simulink model "OrientationAnimationModel"  (R2021b)
settings: Solver=FixedStepAuto  StartTime=0.0  StopTime=1000  FixedStep=.01  RelTol=1e-3
model workspace (MAT data in the model file):
  orbit_altitude = 450000
  r_earth = 6378100
  vel_init = 7640
libraries: matrix_library x5, vrlib x4, aerolibutil x1
settings Model: Creator=Ian Lee  LastModifiedBy=Ian Lee

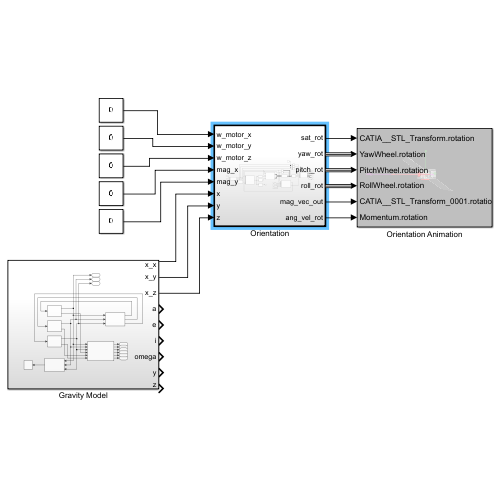
[thumbnail: Simulink's stored preview of the top-level diagram]
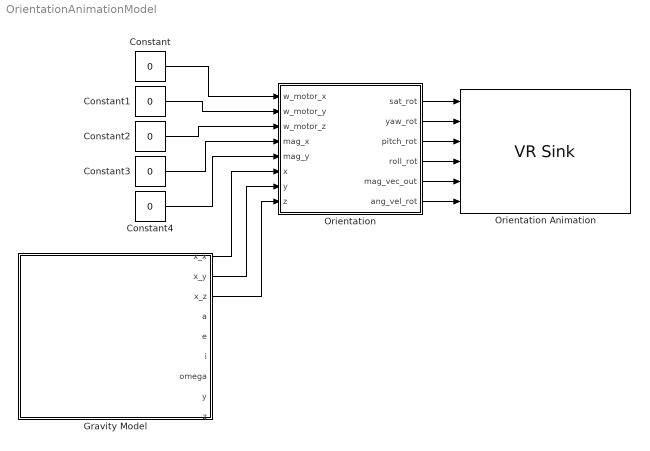
== system OrientationAnimationModel ==
  Constant{,1..4} (5 alike) : Constant  Value=0
  Gravity Model : Subsystem
  Orientation : Subsystem  TreatAsAtomicUnit=on
  Orientation Animation : vrlib/VR Sink  InstantiateOnLoad=on  SampleTime=.02  ViewEnable=on  RemoteChange=off  RemoteView=off  FieldsWritten=CATIA__STL_Transform.rotation.4.1.1.double#YawWheel.rotation.4.1.1.double#PitchWheel.rotation.4.1.1.double#RollWheel.rotation.4.1.1.double#CATIA__STL_Transform_0001.rotation.4.1.1.double#Momentum.rotation.4.1.1.double  WorldFileName=SatVR.x3d  AutoView=off  VideoDimensions=[]  AllowVariableSize=off  FigureProperties="{'Position', 'Name', 'Viewpoint', 'CameraBound', 'CameraDirection', 'CameraPosition', 'CameraUpVector', 'ZoomFactor', 'Antialiasing', 'Headlight', 'Lighting', 'NavPanel', 'Sound', 'StatusBar', 'Stereo3D', 'Stereo3DCameraOffset', 'Stereo3DHIT', 'ToolBar', 'Textures', 'Transparency', 'Triad', 'Wireframe', 'NavZones', 'NavMode', 'NavSpeed', 'CaptureFileFormat', 'CaptureFileName', 'Record2DCompressMethod', 'Record2DCompressQuality', 'Record2D', 'Record2DFileName', 'Record2DFPS'; [1.9340000000000000e+03  -2.3500000000000000e+02   1.0450000000000000e+03   5.1800000000000000e+02], '', '', 'on', [9.3422561981923258e-01  -2.9372272322992476e-01   2.0235971222811577e-01], [-9.5587776533600538e+02   2.6133093944556913e+02  -2.2202783758914998e+02], [2.5834757823765275e-01   9.4839129528426602e-01   1.8387626232948465e-01], [1.0000000000000000e+00], 'on', 'on', 'on', 'halfbar', 'on', 'on', 'off', [1.0000000149011612e-01], [0.0000000000000000e+00], 'on', 'on', 'on', 'none', 'off', 'on', 'examine', 'normal', 'tif', '%f_anim_%n.tif', 'auto', [7.5000000000000000e+01], 'off', '%f_anim_%n.avi', 'auto'}"
  wires:
  Orientation/1(sat_rot) -> Orientation Animation/1
  Orientation/2(yaw_rot) -> Orientation Animation/2
  Orientation/3(pitch_rot) -> Orientation Animation/3
  Orientation/4(roll_rot) -> Orientation Animation/4
  Orientation/5(mag_vec_out) -> Orientation Animation/5
  Orientation/6(ang_vel_rot) -> Orientation Animation/6
  Constant4/1 -> Orientation/5(mag_y)
  Constant3/1 -> Orientation/4(mag_x)
  Constant2/1 -> Orientation/3(w_motor_z)
  Constant1/1 -> Orientation/2(w_motor_y)
  Constant/1 -> Orientation/1(w_motor_x)
  Gravity Model/1(x_x) -> Orientation/6(x)
  Gravity Model/2(x_y) -> Orientation/7(y)
  Gravity Model/3(x_z) -> Orientation/8(z)

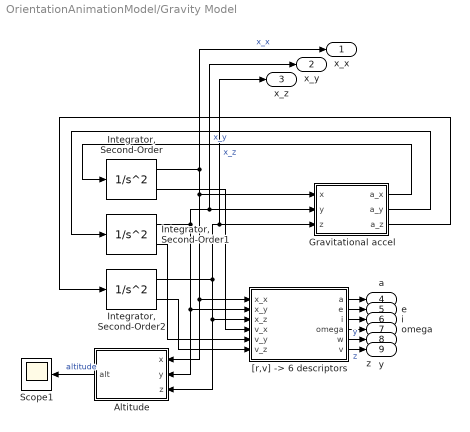
== system OrientationAnimationModel/Gravity Model ==
  Altitude : MATLAB Function  TreatAsAtomicUnit=on
  Gravitational accel : MATLAB Function  TreatAsAtomicUnit=on
  "Integrator, Second-Order" : SecondOrderIntegrator  ICX=0  ICDXDT=5500
  "Integrator, Second-Order1" : SecondOrderIntegrator  ICX=r_earth + orbit_altitude  ICDXDT=0
  "Integrator, Second-Order2" : SecondOrderIntegrator  ICDXDT=5300
  Scope1 : Scope
  "[r,v] -> 6 descriptors" : MATLAB Function  TreatAsAtomicUnit=on
  x_x : Outport
  x_y : Outport  Port=2
  x_z : Outport  Port=3
  a : Outport  Port=4
  e : Outport  Port=5
  i : Outport  Port=6
  omega : Outport  Port=7
  y : Outport  Port=8
  z : Outport  Port=9
  wires:
  Altitude/1(alt) -> Scope1/1  "altitude"
  "Integrator, Second-Order"/1 -> x_x/1, "[r,v] -> 6 descriptors"/1(x_x), Altitude/1(x), Gravitational accel/1(x)  "x_x"
  Gravitational accel/3(a_z) -> "Integrator, Second-Order2"/1
  Gravitational accel/1(a_x) -> "Integrator, Second-Order"/1
  "Integrator, Second-Order1"/1 -> "[r,v] -> 6 descriptors"/2(x_y), Altitude/2(y), x_y/1, Gravitational accel/2(y)  "x_y"
  "Integrator, Second-Order"/2 -> "[r,v] -> 6 descriptors"/4(v_x)
  Gravitational accel/2(a_y) -> "Integrator, Second-Order1"/1
  "Integrator, Second-Order2"/1 -> "[r,v] -> 6 descriptors"/3(x_z), Altitude/3(z), x_z/1, Gravitational accel/3(z)  "x_z"
  "Integrator, Second-Order2"/2 -> "[r,v] -> 6 descriptors"/6(v_z)
  "[r,v] -> 6 descriptors"/4(omega) -> omega/1
  "Integrator, Second-Order1"/2 -> "[r,v] -> 6 descriptors"/5(v_y)
  "[r,v] -> 6 descriptors"/1(a) -> a/1
  "[r,v] -> 6 descriptors"/2(e) -> e/1
  "[r,v] -> 6 descriptors"/5(w) -> y/1  "y"
  "[r,v] -> 6 descriptors"/6(v) -> z/1  "z"
  "[r,v] -> 6 descriptors"/3(i) -> i/1

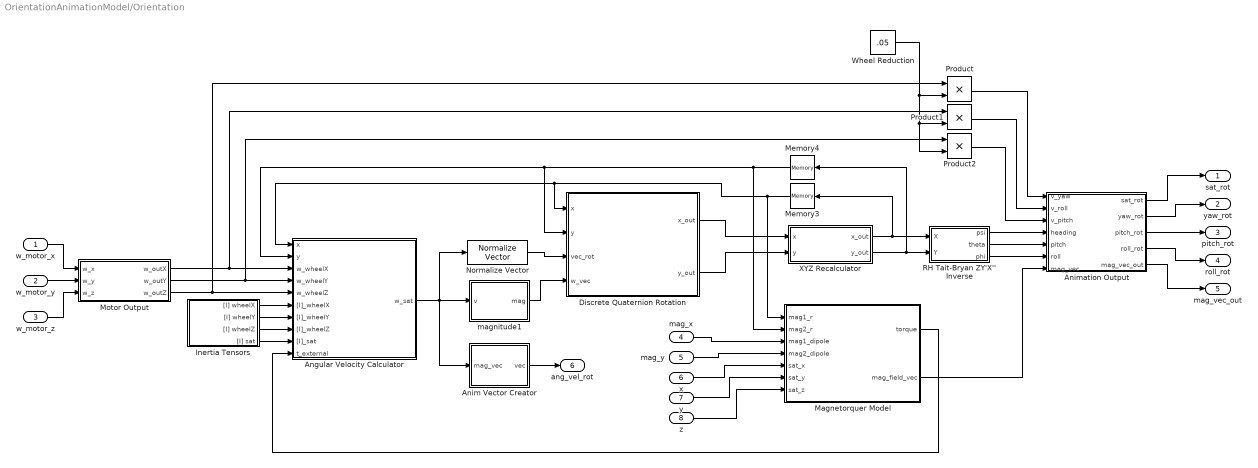
== system OrientationAnimationModel/Orientation ==
  w_motor_x : Inport
  w_motor_y : Inport  Port=2
  w_motor_z : Inport  Port=3
  mag_x : Inport  Port=4
  mag_y : Inport  Port=5
  x : Inport  Port=6
  y : Inport  Port=7
  z : Inport  Port=8
  Angular Velocity Calculator : Subsystem  TreatAsAtomicUnit=on
  Anim Vector Creator : MATLAB Function  TreatAsAtomicUnit=on
  Animation Output : Subsystem  TreatAsAtomicUnit=on
  Discrete Quaternion Rotation : Subsystem  TreatAsAtomicUnit=on
      mask Display: image('C:\Users\benml\Downloads\imageMas.png'); % Use "Edit Image" on toolstrip to change.
  Inertia Tensors : Subsystem  TreatAsAtomicUnit=on
  Magnetorquer Model : Subsystem  TreatAsAtomicUnit=on
  Memory3 : Memory  InitialCondition=[1,0,0]
  Memory4 : Memory  InitialCondition=[0,1,0]
  Motor Output : Subsystem  TreatAsAtomicUnit=on
  Normalize Vector : vrlib/Utilities/Normalize Vector  maxzero=0
  Product : Product
  Product1 : Product
  Product2 : Product
  RH Tait-Bryan ZY'X'' Inverse : MATLAB Function  TreatAsAtomicUnit=on
  Wheel Reduction : Constant  Value=.05
  XYZ Recalculator : Subsystem  TreatAsAtomicUnit=on
  magnitude1 : MATLAB Function  TreatAsAtomicUnit=on
  sat_rot : Outport
  yaw_rot : Outport  Port=2
  pitch_rot : Outport  Port=3
  roll_rot : Outport  Port=4
  mag_vec_out : Outport  Port=5
  ang_vel_rot : Outport  Port=6
  wires:
  Magnetorquer Model/1(torque) -> Angular Velocity Calculator/10(t_external)
  XYZ Recalculator/1(x_out) -> Memory3/1, RH Tait-Bryan ZY'X'' Inverse/1(X)
  RH Tait-Bryan ZY'X'' Inverse/2(theta) -> Animation Output/5(pitch)
  RH Tait-Bryan ZY'X'' Inverse/1(psi) -> Animation Output/4(heading)
  Discrete Quaternion Rotation/1(x_out) -> XYZ Recalculator/1(x)
  Product2/1 -> Animation Output/3(v_pitch)
  Discrete Quaternion Rotation/2(y_out) -> XYZ Recalculator/2(y)
  Product1/1 -> Animation Output/2(v_roll)
  Animation Output/2(yaw_rot) -> yaw_rot/1
  Animation Output/3(pitch_rot) -> pitch_rot/1
  Motor Output/1(w_outX) -> Angular Velocity Calculator/3(w_wheelX), Product1/1
  XYZ Recalculator/2(y_out) -> RH Tait-Bryan ZY'X'' Inverse/2(Y), Memory4/1
  RH Tait-Bryan ZY'X'' Inverse/3(phi) -> Animation Output/6(roll)
  Motor Output/3(w_outZ) -> Angular Velocity Calculator/5(w_wheelZ), Product/1
  Motor Output/2(w_outY) -> Product2/1, Angular Velocity Calculator/4(w_wheelY)
  Animation Output/1(sat_rot) -> sat_rot/1
  Product/1 -> Animation Output/1(v_yaw)
  Memory3/1 -> Magnetorquer Model/1(mag1_r), Discrete Quaternion Rotation/1(x), Angular Velocity Calculator/1(x)
  Animation Output/5(mag_vec_out) -> mag_vec_out/1
  Memory4/1 -> Magnetorquer Model/2(mag2_r), Discrete Quaternion Rotation/2(y), Angular Velocity Calculator/2(y)
  Animation Output/4(roll_rot) -> roll_rot/1
  z/1 -> Magnetorquer Model/7(sat_z)
  y/1 -> Magnetorquer Model/6(sat_y)
  x/1 -> Magnetorquer Model/5(sat_x)
  w_motor_y/1 -> Motor Output/2(w_y)
  w_motor_x/1 -> Motor Output/1(w_x)
  w_motor_z/1 -> Motor Output/3(w_z)
  mag_x/1 -> Magnetorquer Model/3(mag1_dipole)
  mag_y/1 -> Magnetorquer Model/4(mag2_dipole)
  Inertia Tensors/1("[I] wheelX") -> Angular Velocity Calculator/6("[I]_wheelX")
  Inertia Tensors/2("[I] wheelY") -> Angular Velocity Calculator/7("[I]_wheelY")
  Inertia Tensors/3("[I] wheelZ") -> Angular Velocity Calculator/8("[I]_wheelZ")
  Inertia Tensors/4("[I] sat") -> Angular Velocity Calculator/9("[I]_sat")
  Angular Velocity Calculator/1(w_sat) -> Normalize Vector/1, Anim Vector Creator/1(mag_vec), magnitude1/1(v)
  Normalize Vector/1 -> Discrete Quaternion Rotation/3(vec_rot)
  magnitude1/1(mag) -> Discrete Quaternion Rotation/4(w_vec)
  Anim Vector Creator/1(vec) -> ang_vel_rot/1
  Magnetorquer Model/2(mag_field_vec) -> Animation Output/7(mag_vec)
  Wheel Reduction/1 -> Product2/2, Product1/2, Product/2

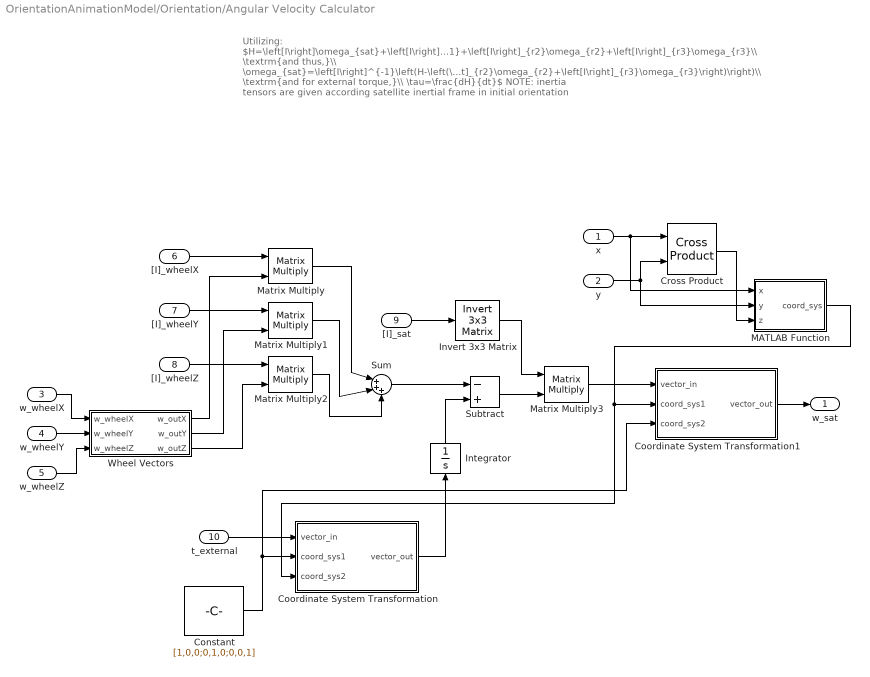
== system OrientationAnimationModel/Orientation/Angular Velocity Calculator ==
  note: Utilizing:
      | $H=\left[I\right]\omega_{sat}+\left[I\right]_{r1}\omega_{r1}+\left[I\right]_{r2}\omega_{r2}+\left[I\right]_{r3}\omega_{r3}\\ \textrm{and thus,}\\ \omega_{sat}=\left[I\right]^{-1}\left(H-\left(\left[I\right]_{r1}\omega_{r1}+\left[I\right]_{r2}\omega_{r2}+\left[I\right]_{r3}\omega_{r3}\right)\right)\\ \textrm{and for external torque,}\\ \tau=\frac{dH}{dt}$
      |
      | NOTE: inertia tensors are given according satellite inertial frame in initial orientation
  x : Inport
  y : Inport  Port=2
  w_wheelX : Inport  Port=3
  w_wheelY : Inport  Port=4
  w_wheelZ : Inport  Port=5
  "[I]_wheelX" : Inport  Port=6
  "[I]_wheelY" : Inport  Port=7
  "[I]_wheelZ" : Inport  Port=8
  "[I]_sat" : Inport  Port=9
  t_external : Inport  Port=10
  Constant : Constant  Value=[1,0,0;0,1,0;0,0,1]
  Coordinate System Transformation : MATLAB Function  TreatAsAtomicUnit=on
  Coordinate System Transformation1 : MATLAB Function  TreatAsAtomicUnit=on
  Cross Product : matrix_library/Cross Product
      settings: SourceProductBaseCode=SL
  Integrator : Integrator
  Invert 3x3 Matrix : aerolibutil/Invert  3x3 Matrix
  MATLAB Function : MATLAB Function  TreatAsAtomicUnit=on
  Matrix Multiply{,1..3} (4 alike) : Product  Multiplication=Matrix(*)
  Subtract : Sum  Inputs=-+
  Sum : Sum  Inputs=|+++
  Wheel Vectors : Subsystem  TreatAsAtomicUnit=on
  w_sat : Outport
  wires:
  "[I]_sat"/1 -> Invert 3x3 Matrix/1
  w_wheelX/1 -> Wheel Vectors/1(w_wheelX)
  w_wheelY/1 -> Wheel Vectors/2(w_wheelY)
  w_wheelZ/1 -> Wheel Vectors/3(w_wheelZ)
  "[I]_wheelX"/1 -> Matrix Multiply/1
  "[I]_wheelY"/1 -> Matrix Multiply1/1
  "[I]_wheelZ"/1 -> Matrix Multiply2/1
  Wheel Vectors/1(w_outX) -> Matrix Multiply/2
  Wheel Vectors/2(w_outY) -> Matrix Multiply1/2
  Wheel Vectors/3(w_outZ) -> Matrix Multiply2/2
  Matrix Multiply1/1 -> Sum/2
  Matrix Multiply2/1 -> Sum/3
  Matrix Multiply/1 -> Sum/1
  Invert 3x3 Matrix/1 -> Matrix Multiply3/1
  x/1 -> MATLAB Function/1(x), Cross Product/1
  y/1 -> MATLAB Function/2(y), Cross Product/2
  Cross Product/1 -> MATLAB Function/3(z)
  MATLAB Function/1(coord_sys) -> Coordinate System Transformation/3(coord_sys2), Coordinate System Transformation1/2(coord_sys1)
  Subtract/1 -> Matrix Multiply3/2
  t_external/1 -> Coordinate System Transformation/1(vector_in)
  Sum/1 -> Subtract/1
  Constant/1 -> Coordinate System Transformation/2(coord_sys1), Coordinate System Transformation1/3(coord_sys2)
  Matrix Multiply3/1 -> Coordinate System Transformation1/1(vector_in)
  Coordinate System Transformation1/1(vector_out) -> w_sat/1
  Coordinate System Transformation/1(vector_out) -> Integrator/1
  Integrator/1 -> Subtract/2

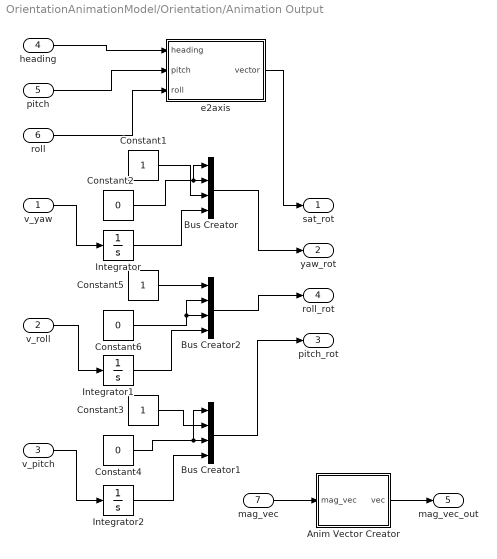
== system OrientationAnimationModel/Orientation/Animation Output ==
  v_yaw : Inport
  v_roll : Inport  Port=2
  v_pitch : Inport  Port=3
  heading : Inport  Port=4
  pitch : Inport  Port=5
  roll : Inport  Port=6
  mag_vec : Inport  Port=7
  Anim Vector Creator : MATLAB Function  TreatAsAtomicUnit=on
  Bus Creator : BusCreator  Inputs=4
  Bus Creator1 : BusCreator  Inputs=4
  Bus Creator2 : BusCreator  Inputs=4
  Constant1 : Constant
  Constant2 : Constant  Value=0
  Constant3 : Constant
  Constant4 : Constant  Value=0
  Constant5 : Constant
  Constant6 : Constant  Value=0
  Integrator : Integrator
  Integrator1 : Integrator
  Integrator2 : Integrator
  e2axis : MATLAB Function  TreatAsAtomicUnit=on
  sat_rot : Outport
  yaw_rot : Outport  Port=2
  pitch_rot : Outport  Port=3
  roll_rot : Outport  Port=4
  mag_vec_out : Outport  Port=5
  wires:
  Constant6/1 -> Bus Creator2/2, Bus Creator2/3
  Constant5/1 -> Bus Creator2/1
  Constant1/1 -> Bus Creator/3
  Constant3/1 -> Bus Creator1/2
  Constant2/1 -> Bus Creator/1, Bus Creator/2
  Constant4/1 -> Bus Creator1/1, Bus Creator1/3
  heading/1 -> e2axis/1(heading)
  pitch/1 -> e2axis/2(pitch)
  roll/1 -> e2axis/3(roll)
  e2axis/1(vector) -> sat_rot/1
  v_yaw/1 -> Integrator/1
  v_roll/1 -> Integrator1/1
  v_pitch/1 -> Integrator2/1
  Bus Creator/1 -> yaw_rot/1
  Bus Creator2/1 -> roll_rot/1
  Bus Creator1/1 -> pitch_rot/1
  Integrator/1 -> Bus Creator/4
  Integrator1/1 -> Bus Creator2/4
  Integrator2/1 -> Bus Creator1/4
  mag_vec/1 -> Anim Vector Creator/1(mag_vec)
  Anim Vector Creator/1(vec) -> mag_vec_out/1

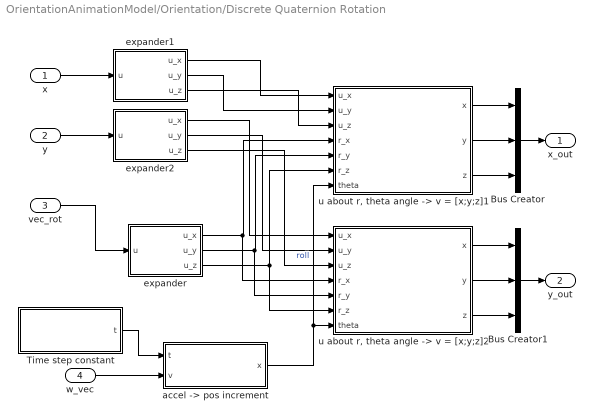
== system OrientationAnimationModel/Orientation/Discrete Quaternion Rotation ==
  x : Inport
  y : Inport  Port=2
  vec_rot : Inport  Port=3
  w_vec : Inport  Port=4
  Bus Creator : BusCreator  Inputs=3
  Bus Creator1 : BusCreator  Inputs=3
  Time step constant : Subsystem  TreatAsAtomicUnit=on
  "accel -> pos increment" : Subsystem  TreatAsAtomicUnit=on
  expander : MATLAB Function  TreatAsAtomicUnit=on
  expander1 : MATLAB Function  TreatAsAtomicUnit=on
  expander2 : MATLAB Function  TreatAsAtomicUnit=on
  "u about r, theta angle -> v = [x;y;z]1" : Subsystem  TreatAsAtomicUnit=on
  "u about r, theta angle -> v = [x;y;z]2" : Subsystem  TreatAsAtomicUnit=on
  x_out : Outport
  y_out : Outport  Port=2
  wires:
  x/1 -> expander1/1(u)
  vec_rot/1 -> expander/1(u)
  expander1/1(u_x) -> "u about r, theta angle -> v = [x;y;z]1"/1(u_x)
  expander1/2(u_y) -> "u about r, theta angle -> v = [x;y;z]1"/2(u_y)
  expander1/3(u_z) -> "u about r, theta angle -> v = [x;y;z]1"/3(u_z)
  expander/1(u_x) -> "u about r, theta angle -> v = [x;y;z]2"/4(r_x), "u about r, theta angle -> v = [x;y;z]1"/4(r_x)
  expander/2(u_y) -> "u about r, theta angle -> v = [x;y;z]2"/5(r_y), "u about r, theta angle -> v = [x;y;z]1"/5(r_y)
  expander/3(u_z) -> "u about r, theta angle -> v = [x;y;z]1"/6(r_z), "u about r, theta angle -> v = [x;y;z]2"/6(r_z)
  expander2/1(u_x) -> "u about r, theta angle -> v = [x;y;z]2"/1(u_x)
  expander2/2(u_y) -> "u about r, theta angle -> v = [x;y;z]2"/2(u_y)
  expander2/3(u_z) -> "u about r, theta angle -> v = [x;y;z]2"/3(u_z)
  y/1 -> expander2/1(u)
  Time step constant/1(t) -> "accel -> pos increment"/1(t)
  "accel -> pos increment"/1(x) -> "u about r, theta angle -> v = [x;y;z]1"/7(theta), "u about r, theta angle -> v = [x;y;z]2"/7(theta)  "roll"
  w_vec/1 -> "accel -> pos increment"/2("v ")
  "u about r, theta angle -> v = [x;y;z]1"/1(x) -> Bus Creator/1
  "u about r, theta angle -> v = [x;y;z]1"/2(y) -> Bus Creator/2
  "u about r, theta angle -> v = [x;y;z]1"/3(z) -> Bus Creator/3
  Bus Creator/1 -> x_out/1
  Bus Creator1/1 -> y_out/1
  "u about r, theta angle -> v = [x;y;z]2"/2(y) -> Bus Creator1/2
  "u about r, theta angle -> v = [x;y;z]2"/1(x) -> Bus Creator1/1
  "u about r, theta angle -> v = [x;y;z]2"/3(z) -> Bus Creator1/3

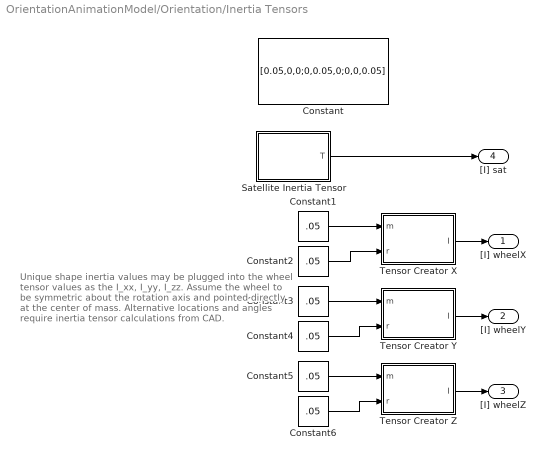
== system OrientationAnimationModel/Orientation/Inertia Tensors ==
  note: Unique shape inertia values may be plugged into
      | the wheel tensor values as the I_xx, I_yy, I_zz. Assume
      | the wheel to be symmetric about the rotation axis
      | and pointed directly at the center of mass.
      | Alternative locations and angles require inertia
      | tensor calculations from CAD.
  Constant : Constant  Value=[0.05,0,0;0,0.05,0;0,0,0.05]
  Constant{1..6} (6 alike) : Constant  Value=.05
  Satellite Inertia Tensor : MATLAB Function  TreatAsAtomicUnit=on
  Tensor Creator X : MATLAB Function  TreatAsAtomicUnit=on
  Tensor Creator Y : MATLAB Function  TreatAsAtomicUnit=on
  Tensor Creator Z : MATLAB Function  TreatAsAtomicUnit=on
  "[I] wheelX" : Outport
  "[I] wheelY" : Outport  Port=2
  "[I] wheelZ" : Outport  Port=3
  "[I] sat" : Outport  Port=4
  wires:
  Constant2/1 -> Tensor Creator X/2(r)
  Constant1/1 -> Tensor Creator X/1(m)
  Constant4/1 -> Tensor Creator Y/2(r)
  Constant3/1 -> Tensor Creator Y/1(m)
  Constant6/1 -> Tensor Creator Z/2(r)
  Constant5/1 -> Tensor Creator Z/1(m)
  Tensor Creator Y/1(I) -> "[I] wheelY"/1
  Tensor Creator X/1(I) -> "[I] wheelX"/1
  Tensor Creator Z/1(I) -> "[I] wheelZ"/1
  Satellite Inertia Tensor/1(T) -> "[I] sat"/1

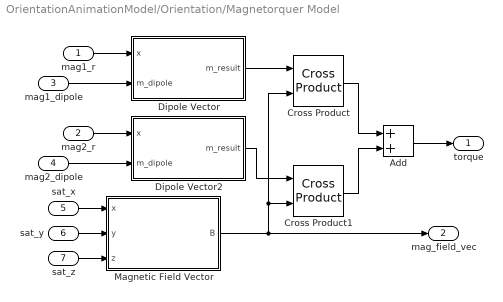
== system OrientationAnimationModel/Orientation/Magnetorquer Model ==
  mag1_r : Inport
  mag2_r : Inport  Port=2
  mag1_dipole : Inport  Port=3
  mag2_dipole : Inport  Port=4
  sat_x : Inport  Port=5
  sat_y : Inport  Port=6
  sat_z : Inport  Port=7
  Add : Sum
  Cross Product : matrix_library/Cross Product
      settings: SourceProductBaseCode=SL
  Cross Product1 : matrix_library/Cross Product
      settings: SourceProductBaseCode=SL
  Dipole Vector : MATLAB Function  TreatAsAtomicUnit=on
  Dipole Vector2 : MATLAB Function  TreatAsAtomicUnit=on
  Magnetic Field Vector : MATLAB Function  TreatAsAtomicUnit=on
  torque : Outport
  mag_field_vec : Outport  Port=2
  wires:
  Cross Product1/1 -> Add/2
  mag1_dipole/1 -> Dipole Vector/2(m_dipole)
  Cross Product/1 -> Add/1
  Dipole Vector2/1(m_result) -> Cross Product1/1
  sat_x/1 -> Magnetic Field Vector/1(x)
  sat_z/1 -> Magnetic Field Vector/3(z)
  sat_y/1 -> Magnetic Field Vector/2(y)
  Magnetic Field Vector/1(B) -> mag_field_vec/1, Cross Product/2, Cross Product1/2
  mag2_dipole/1 -> Dipole Vector2/2(m_dipole)
  Dipole Vector/1(m_result) -> Cross Product/1
  Add/1 -> torque/1
  mag2_r/1 -> Dipole Vector2/1(x)
  mag1_r/1 -> Dipole Vector/1(x)

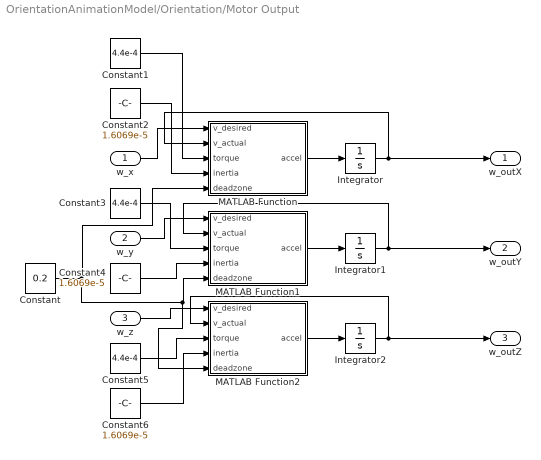
== system OrientationAnimationModel/Orientation/Motor Output ==
  w_x : Inport
  w_y : Inport  Port=2
  w_z : Inport  Port=3
  Constant : Constant  Value=0.2
  Constant1 : Constant  Value=4.4e-4
  Constant2 : Constant  Value=1.6069e-5
  Constant3 : Constant  Value=4.4e-4
  Constant4 : Constant  Value=1.6069e-5
  Constant5 : Constant  Value=4.4e-4
  Constant6 : Constant  Value=1.6069e-5
  Integrator : Integrator
  Integrator1 : Integrator
  Integrator2 : Integrator
  MATLAB Function : MATLAB Function  TreatAsAtomicUnit=on
  MATLAB Function1 : MATLAB Function  TreatAsAtomicUnit=on
  MATLAB Function2 : MATLAB Function  TreatAsAtomicUnit=on
  w_outX : Outport
  w_outY : Outport  Port=2
  w_outZ : Outport  Port=3
  wires:
  Constant1/1 -> MATLAB Function/3(torque)
  Constant2/1 -> MATLAB Function/4(inertia)
  MATLAB Function/1(accel) -> Integrator/1
  Integrator/1 -> MATLAB Function/2(v_actual), w_outX/1
  w_x/1 -> MATLAB Function/1(v_desired)
  Constant3/1 -> MATLAB Function1/3(torque)
  Constant4/1 -> MATLAB Function1/4(inertia)
  MATLAB Function1/1(accel) -> Integrator1/1
  Integrator1/1 -> w_outY/1, MATLAB Function1/2(v_actual)
  w_y/1 -> MATLAB Function1/1(v_desired)
  Constant5/1 -> MATLAB Function2/3(torque)
  Constant6/1 -> MATLAB Function2/4(inertia)
  MATLAB Function2/1(accel) -> Integrator2/1
  Integrator2/1 -> MATLAB Function2/2(v_actual), w_outZ/1
  w_z/1 -> MATLAB Function2/1(v_desired)
  Constant/1 -> MATLAB Function2/5(deadzone), MATLAB Function1/5(deadzone), MATLAB Function/5(deadzone)

== system OrientationAnimationModel/Orientation/XYZ Recalculator ==
  x : Inport
  y : Inport  Port=2
  Cross Product : matrix_library/Cross Product
      settings: SourceProductBaseCode=SL
  Cross Product1 : matrix_library/Cross Product
      settings: SourceProductBaseCode=SL
  Normalize Vector : vrlib/Utilities/Normalize Vector  maxzero=0
  Normalize Vector1 : vrlib/Utilities/Normalize Vector  maxzero=0
  x_out : Outport
  y_out : Outport  Port=2
  wires:
  x/1 -> Normalize Vector1/1
  y/1 -> y_out/1, Cross Product1/1, Normalize Vector/1
  Normalize Vector1/1 -> Cross Product/1
  Normalize Vector/1 -> Cross Product/2
  Cross Product/1 -> Cross Product1/2
  Cross Product1/1 -> x_out/1

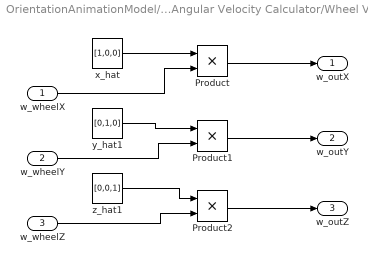
== system OrientationAnimationModel/Orientation/Angular Velocity Calculator/Wheel Vectors ==
  w_wheelX : Inport
  w_wheelY : Inport  Port=2
  w_wheelZ : Inport  Port=3
  Product : Product
  Product1 : Product
  Product2 : Product
  x_hat : Constant  Value=[1,0,0]
  y_hat1 : Constant  Value=[0,1,0]
  z_hat1 : Constant  Value=[0,0,1]
  w_outX : Outport
  w_outY : Outport  Port=2
  w_outZ : Outport  Port=3
  wires:
  x_hat/1 -> Product/1
  w_wheelX/1 -> Product/2
  y_hat1/1 -> Product1/1
  z_hat1/1 -> Product2/1
  w_wheelY/1 -> Product1/2
  w_wheelZ/1 -> Product2/2
  Product/1 -> w_outX/1
  Product1/1 -> w_outY/1
  Product2/1 -> w_outZ/1

== system OrientationAnimationModel/Orientation/Discrete Quaternion Rotation/Time step constant ==
  Clock : Clock
  Memory : Memory  InitialCondition=0.1
  Subtract : Sum  Inputs=+-
  t : Outport
  wires:
  Clock/1 -> Memory/1, Subtract/1
  Memory/1 -> Subtract/2
  Subtract/1 -> t/1

== system OrientationAnimationModel/Orientation/Discrete Quaternion Rotation/accel -> pos increment ==
  t : Inport
  "v " : Inport  Port=2
  Gain : Gain
  Product : Product
  x : Outport
  wires:
  t/1 -> Product/1
  "v "/1 -> Product/2
  Product/1 -> Gain/1
  Gain/1 -> x/1

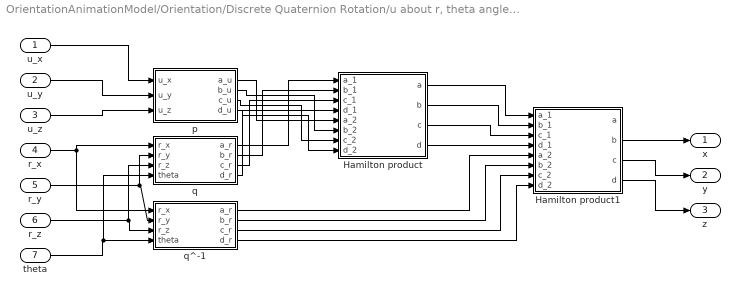
== system OrientationAnimationModel/Orientation/Discrete Quaternion Rotation/u about r, theta angle -> v = [x;y;z]1 ==
  u_x : Inport
  u_y : Inport  Port=2
  u_z : Inport  Port=3
  r_x : Inport  Port=4
  r_y : Inport  Port=5
  r_z : Inport  Port=6
  theta : Inport  Port=7
  Hamilton product : MATLAB Function  TreatAsAtomicUnit=on
  Hamilton product1 : MATLAB Function  TreatAsAtomicUnit=on
  p : MATLAB Function  TreatAsAtomicUnit=on
  q : MATLAB Function  TreatAsAtomicUnit=on
  q^-1 : MATLAB Function  TreatAsAtomicUnit=on
  x : Outport
  y : Outport  Port=2
  z : Outport  Port=3
  wires:
  Hamilton product/1(a) -> Hamilton product1/1(a_1)
  Hamilton product/2(b) -> Hamilton product1/2(b_1)
  Hamilton product/3(c) -> Hamilton product1/3(c_1)
  Hamilton product/4(d) -> Hamilton product1/4(d_1)
  q^-1/1(a_r) -> Hamilton product1/5(a_2)
  q^-1/2(b_r) -> Hamilton product1/6(b_2)
  q^-1/3(c_r) -> Hamilton product1/7(c_2)
  q^-1/4(d_r) -> Hamilton product1/8(d_2)
  theta/1 -> q/4(theta), q^-1/4(theta)
  r_z/1 -> q/3(r_z), q^-1/3(r_z)
  r_y/1 -> q/2(r_y), q^-1/2(r_y)
  r_x/1 -> q/1(r_x), q^-1/1(r_x)
  u_z/1 -> p/3(u_z)
  u_y/1 -> p/2(u_y)
  u_x/1 -> p/1(u_x)
  Hamilton product1/2(b) -> x/1
  Hamilton product1/3(c) -> y/1
  Hamilton product1/4(d) -> z/1
  q/1(a_r) -> Hamilton product/1(a_1)
  q/2(b_r) -> Hamilton product/2(b_1)
  q/3(c_r) -> Hamilton product/3(c_1)
  q/4(d_r) -> Hamilton product/4(d_1)
  p/2(b_u) -> Hamilton product/6(b_2)
  p/3(c_u) -> Hamilton product/7(c_2)
  p/4(d_u) -> Hamilton product/8(d_2)
  p/1(a_u) -> Hamilton product/5(a_2)

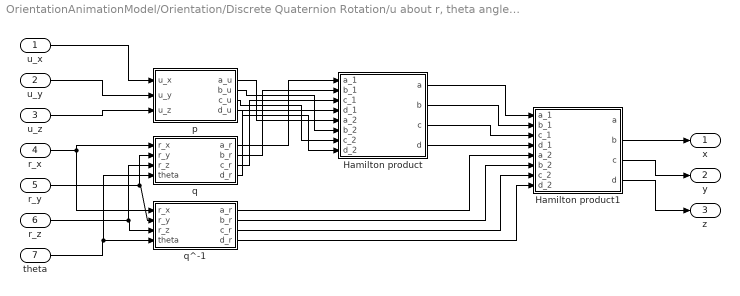
== system OrientationAnimationModel/Orientation/Discrete Quaternion Rotation/u about r, theta angle -> v = [x;y;z]2 ==
  u_x : Inport
  u_y : Inport  Port=2
  u_z : Inport  Port=3
  r_x : Inport  Port=4
  r_y : Inport  Port=5
  r_z : Inport  Port=6
  theta : Inport  Port=7
  Hamilton product : MATLAB Function  TreatAsAtomicUnit=on
  Hamilton product1 : MATLAB Function  TreatAsAtomicUnit=on
  p : MATLAB Function  TreatAsAtomicUnit=on
  q : MATLAB Function  TreatAsAtomicUnit=on
  q^-1 : MATLAB Function  TreatAsAtomicUnit=on
  x : Outport
  y : Outport  Port=2
  z : Outport  Port=3
  wires:
  Hamilton product/1(a) -> Hamilton product1/1(a_1)
  Hamilton product/2(b) -> Hamilton product1/2(b_1)
  Hamilton product/3(c) -> Hamilton product1/3(c_1)
  Hamilton product/4(d) -> Hamilton product1/4(d_1)
  q^-1/1(a_r) -> Hamilton product1/5(a_2)
  q^-1/2(b_r) -> Hamilton product1/6(b_2)
  q^-1/3(c_r) -> Hamilton product1/7(c_2)
  q^-1/4(d_r) -> Hamilton product1/8(d_2)
  theta/1 -> q/4(theta), q^-1/4(theta)
  r_z/1 -> q/3(r_z), q^-1/3(r_z)
  r_y/1 -> q/2(r_y), q^-1/2(r_y)
  r_x/1 -> q/1(r_x), q^-1/1(r_x)
  u_z/1 -> p/3(u_z)
  u_y/1 -> p/2(u_y)
  u_x/1 -> p/1(u_x)
  Hamilton product1/2(b) -> x/1
  Hamilton product1/3(c) -> y/1
  Hamilton product1/4(d) -> z/1
  q/1(a_r) -> Hamilton product/1(a_1)
  q/2(b_r) -> Hamilton product/2(b_1)
  q/3(c_r) -> Hamilton product/3(c_1)
  q/4(d_r) -> Hamilton product/4(d_1)
  p/2(b_u) -> Hamilton product/6(b_2)
  p/3(c_u) -> Hamilton product/7(c_2)
  p/4(d_u) -> Hamilton product/8(d_2)
  p/1(a_u) -> Hamilton product/5(a_2)

== matlab function OrientationAnimationModel/Orientation/Angular Velocity Calculator/MATLAB Function ==
  data: x input; coord_sys output; y input; z input
function coord_sys = fcn(x,y,z)

coord_sys = [x(1),x(2),x(3);y(1),y(2),y(3);z(1),z(2),z(3)];

== matlab function OrientationAnimationModel/Orientation/Discrete Quaternion Rotation/expander ==
  data: u input; u_x output; u_y output; u_z output
function [u_x,u_y,u_z] = fcn(u)

u_x = u(1);
u_y = u(2);
u_z = u(3);

== matlab function OrientationAnimationModel/Orientation/Inertia Tensors/Satellite Inertia Tensor ==
  data: T output
function T = fcn

T = [
0.04, 0.00, 0.00;
0.00, 0.05, 0.02;
0.00, 0.02, 0.05
];

== matlab function OrientationAnimationModel/Orientation/Angular Velocity Calculator/Coordinate System Transformation ==
  data: vector_in input; vector_out output; coord_sys1 input; coord_sys2 input
% transform tensor from standard cartesian to another given rotated cartesian system unit
% vectors
function vector_out = fcn(vector_in,coord_sys1,coord_sys2)

% normalize coordinate systems
coord_sys1 = coord_sys1 / norm(coord_sys1);
coord_sys2 = coord_sys2 / norm(coord_sys2);

c2 = coord_sys2;
c1 = coord_sys1;

trans_mat = [
dot(c2(1,:),c1(1,:)), dot(c2(1,:),c1(2,:)), dot(c2(1,:),c1(3,:));
dot(c2(2,:),c1(1,:)), dot(c2(2,:),c1(2,:)), dot(c2(2,:),c1(3,:));
dot(c2(3,:),c1(1,:)), dot(c2(3,:),c1(2,:)), dot(c2(3,:),c1(3,:));
];

vector_out = trans_mat * vector_in;

== matlab function OrientationAnimationModel/Orientation/magnitude1 ==
  data: v input; mag output
function mag = fcn(v)

mag = sqrt(v(1)^2+v(2)^2+v(3)^2);

== matlab function OrientationAnimationModel/Orientation/Inertia Tensors/Tensor Creator X ==
  data: m input; I output; r input
function I = fcn(m,r)

I_xx = 0.5 * m * r^2;
I = [
I_xx, 0, 0;
0, 0, 0;
0, 0, 0;
];

== matlab function OrientationAnimationModel/Orientation/Discrete Quaternion Rotation/expander1 ==
  data: u input; u_x output; u_y output; u_z output
function [u_x,u_y,u_z] = fcn(u)

u_x = u(1);
u_y = u(2);
u_z = u(3);

== matlab function OrientationAnimationModel/Orientation/Discrete Quaternion Rotation/expander2 ==
  data: u input; u_x output; u_y output; u_z output
function [u_x,u_y,u_z] = fcn(u)

u_x = u(1);
u_y = u(2);
u_z = u(3);

== matlab function OrientationAnimationModel/Orientation/Inertia Tensors/Tensor Creator Y ==
  data: m input; I output; r input
function I = fcn(m,r)

I_yy = 0.5 * m * r^2;
I = [
0, 0, 0;
0, I_yy, 0;
0, 0, 0;
];

== matlab function OrientationAnimationModel/Orientation/Inertia Tensors/Tensor Creator Z ==
  data: m input; I output; r input
function I = fcn(m,r)

I_zz = 0.5 * m * r^2;
I = [
0, 0, 0;
0, 0, 0;
0, 0, I_zz;
];

== matlab function OrientationAnimationModel/Orientation/Discrete Quaternion Rotation/u about r, theta angle -> v = [x;y;z]1/Hamilton product ==
  data: a_1 input; a output; b_1 input; c_1 input; d_1 input; a_2 input; b_2 input; c_2 input; d_2 input; b output; c output; d output
function [a, b, c, d] = fcn(a_1, b_1, c_1, d_1, a_2, b_2, c_2, d_2)

a = a_1 * a_2 - b_1 * b_2 - c_1 * c_2 - d_1 * d_2;
b = a_1 * b_2 + b_1 * a_2 + c_1 * d_2 - d_1 * c_2;
c = a_1 * c_2 - b_1 * d_2 + c_1 * a_2 + d_1 * b_2;
d = a_1 * d_2 + b_1 * c_2 - c_1 * b_2 + d_1 * a_2;

== matlab function OrientationAnimationModel/Orientation/Discrete Quaternion Rotation/u about r, theta angle -> v = [x;y;z]1/Hamilton product1 ==
  data: a_1 input; a output; b_1 input; c_1 input; d_1 input; a_2 input; b_2 input; c_2 input; d_2 input; b output; c output; d output
function [a, b, c, d] = fcn(a_1, b_1, c_1, d_1, a_2, b_2, c_2, d_2)

a = a_1 * a_2 - b_1 * b_2 - c_1 * c_2 - d_1 * d_2;
b = a_1 * b_2 + b_1 * a_2 + c_1 * d_2 - d_1 * c_2;
c = a_1 * c_2 - b_1 * d_2 + c_1 * a_2 + d_1 * b_2;
d = a_1 * d_2 + b_1 * c_2 - c_1 * b_2 + d_1 * a_2;

== matlab function OrientationAnimationModel/Orientation/Discrete Quaternion Rotation/u about r, theta angle -> v = [x;y;z]1/p ==
  data: u_x input; u_y input; u_z input; a_u output; b_u output; c_u output; d_u output
function [a_u, b_u, c_u, d_u] = fcn(u_x, u_y, u_z)
a_u = 0;
b_u = u_x;
c_u = u_y;
d_u = u_z;

== matlab function OrientationAnimationModel/Gravity Model/Gravitational accel ==
  data: x input; a_x output; y input; z input; a_y output; a_z output
function [a_x, a_y, a_z] = fcn(x, y, z)
% determine acceleration
d = sqrt(x^2 + y^2 + z^2);
a = -((6.67408*10^-11) * (5.97219*10^24)) / d^2;
% x,y,z unit vector for direction
x1 = x / d;
y1 = y / d;
z1 = z / d;
% x,y,z acceleration vectors
a_x = a * x1;
a_y = a * y1;
a_z = a * z1;

== matlab function OrientationAnimationModel/Orientation/Discrete Quaternion Rotation/u about r, theta angle -> v = [x;y;z]1/q ==
  data: r_x input; a_r output; r_y input; r_z input; theta input; b_r output; c_r output; d_r output
function [a_r, b_r, c_r, d_r] = fcn(r_x, r_y, r_z, theta)

a_r = cos(theta / 2);
b_r = r_x * sin(theta / 2);
c_r = r_y * sin(theta / 2);
d_r = r_z * sin(theta / 2);

== matlab function OrientationAnimationModel/Orientation/Angular Velocity Calculator/Coordinate System Transformation1 ==
  data: vector_in input; vector_out output; coord_sys1 input; coord_sys2 input
% transform tensor from standard cartesian to another given rotated cartesian system unit
% vectors
function vector_out = fcn(vector_in,coord_sys1,coord_sys2)

% normalize coordinate systems
coord_sys1 = coord_sys1 / norm(coord_sys1);
coord_sys2 = coord_sys2 / norm(coord_sys2);

c2 = coord_sys2;
c1 = coord_sys1;

trans_mat = [
dot(c2(1,:),c1(1,:)), dot(c2(1,:),c1(2,:)), dot(c2(1,:),c1(3,:));
dot(c2(2,:),c1(1,:)), dot(c2(2,:),c1(2,:)), dot(c2(2,:),c1(3,:));
dot(c2(3,:),c1(1,:)), dot(c2(3,:),c1(2,:)), dot(c2(3,:),c1(3,:));
];

vector_out = trans_mat * vector_in;

== matlab function OrientationAnimationModel/Orientation/Discrete Quaternion Rotation/u about r, theta angle -> v = [x;y;z]1/q^-1 ==
  data: r_x input; a_r output; r_y input; r_z input; theta input; b_r output; c_r output; d_r output
function [a_r, b_r, c_r, d_r] = fcn(r_x, r_y, r_z, theta)

a_r = cos(theta / 2);
b_r = r_x * -sin(theta / 2);
c_r = r_y * -sin(theta / 2);
d_r = r_z * -sin(theta / 2);

== matlab function OrientationAnimationModel/Orientation/Discrete Quaternion Rotation/u about r, theta angle -> v = [x;y;z]2/Hamilton product ==
  data: a_1 input; a output; b_1 input; c_1 input; d_1 input; a_2 input; b_2 input; c_2 input; d_2 input; b output; c output; d output
function [a, b, c, d] = fcn(a_1, b_1, c_1, d_1, a_2, b_2, c_2, d_2)

a = a_1 * a_2 - b_1 * b_2 - c_1 * c_2 - d_1 * d_2;
b = a_1 * b_2 + b_1 * a_2 + c_1 * d_2 - d_1 * c_2;
c = a_1 * c_2 - b_1 * d_2 + c_1 * a_2 + d_1 * b_2;
d = a_1 * d_2 + b_1 * c_2 - c_1 * b_2 + d_1 * a_2;

== matlab function OrientationAnimationModel/Orientation/Discrete Quaternion Rotation/u about r, theta angle -> v = [x;y;z]2/Hamilton product1 ==
  data: a_1 input; a output; b_1 input; c_1 input; d_1 input; a_2 input; b_2 input; c_2 input; d_2 input; b output; c output; d output
function [a, b, c, d] = fcn(a_1, b_1, c_1, d_1, a_2, b_2, c_2, d_2)

a = a_1 * a_2 - b_1 * b_2 - c_1 * c_2 - d_1 * d_2;
b = a_1 * b_2 + b_1 * a_2 + c_1 * d_2 - d_1 * c_2;
c = a_1 * c_2 - b_1 * d_2 + c_1 * a_2 + d_1 * b_2;
d = a_1 * d_2 + b_1 * c_2 - c_1 * b_2 + d_1 * a_2;

== matlab function OrientationAnimationModel/Orientation/Discrete Quaternion Rotation/u about r, theta angle -> v = [x;y;z]2/p ==
  data: u_x input; u_y input; u_z input; a_u output; b_u output; c_u output; d_u output
function [a_u, b_u, c_u, d_u] = fcn(u_x, u_y, u_z)
a_u = 0;
b_u = u_x;
c_u = u_y;
d_u = u_z;

== matlab function OrientationAnimationModel/Orientation/Discrete Quaternion Rotation/u about r, theta angle -> v = [x;y;z]2/q ==
  data: r_x input; a_r output; r_y input; r_z input; theta input; b_r output; c_r output; d_r output
function [a_r, b_r, c_r, d_r] = fcn(r_x, r_y, r_z, theta)

a_r = cos(theta / 2);
b_r = r_x * sin(theta / 2);
c_r = r_y * sin(theta / 2);
d_r = r_z * sin(theta / 2);

== matlab function OrientationAnimationModel/Orientation/Discrete Quaternion Rotation/u about r, theta angle -> v = [x;y;z]2/q^-1 ==
  data: r_x input; a_r output; r_y input; r_z input; theta input; b_r output; c_r output; d_r output
function [a_r, b_r, c_r, d_r] = fcn(r_x, r_y, r_z, theta)

a_r = cos(theta / 2);
b_r = r_x * -sin(theta / 2);
c_r = r_y * -sin(theta / 2);
d_r = r_z * -sin(theta / 2);

== matlab function OrientationAnimationModel/Gravity Model/[r,v] -> 6 descriptors ==
  data: x_x input; a output; x_y input; x_z input; v_x input; v_y input; v_z input; e output; i output; omega output; w output; v output
function [a, e, i, omega, w, v] = fcn(x_x, x_y, x_z, v_x, v_y, v_z)

% by math magic, we know (SEE RESEARCH FILES\Orbital mechanics.pdf):
% e is the eccentricity vector, that points from apoapsis to periapsis with
% magnitude = orbit's scalar eccentricity; mu is standard gravitational
% parameter: mu = G(m1 + m2), in this case satellite mass is negligible. 

r = [x_x, x_y, x_z];
r_hat = r / norm(r);
r_dot = [v_x, v_y, v_z];
h = cross(r,r_dot);
mu = 3.986004418*10^14;
ecc_vec = (1 / mu) * (cross(r_dot,h) - mu * r_hat);
e = norm(ecc_vec); % e

i = acos(h(3) / norm(h)); % i

spec_mech_e = ((norm(r_dot))^2 / 2) - mu / norm(r);
a = (-mu) / (2 * spec_mech_e); % a

if(i ~= 0)
    n = cross([0,0,1],h);
    omega = acos(n(1) / norm(n)); % omega
    if(n(2) < 0)
        omega = 2*pi - omega;
    end
    
    w = acos(dot(n,ecc_vec) / (norm(n) * e)); % w
    if(ecc_vec(3) < 0)
        w = 2*pi - w;
    end
    
    v = acos(dot(ecc_vec,r) / (norm(r) * e)); % v
    if(dot(r,r_dot) < 0)
        w = 2*pi - w;
    end
else
    omega = 0;
    w = 0;
    v = 0;
end

== matlab function OrientationAnimationModel/Orientation/Anim Vector Creator ==
  data: mag_vec input; vec output
function vec = fcn(mag_vec)

cos_theta = mag_vec(3) / sqrt(mag_vec(1)^2+mag_vec(2)^2+mag_vec(3)^2);
theta = acos(cos_theta);
vec = [-mag_vec(2); mag_vec(1); 0; theta];

== matlab function OrientationAnimationModel/Orientation/Motor Output/MATLAB Function ==
  data: v_desired input; accel output; v_actual input; torque input; inertia input; deadzone input
function accel  = fcn(v_desired, v_actual, torque, inertia, deadzone)
if(v_desired - deadzone > v_actual)
    accel = torque / inertia;
elseif(v_desired + deadzone < v_actual)
    accel = -torque / inertia;
else
    accel = 0;
end

== matlab function OrientationAnimationModel/Orientation/Motor Output/MATLAB Function1 ==
  data: v_desired input; accel output; v_actual input; torque input; inertia input; deadzone input
function accel  = fcn(v_desired, v_actual, torque, inertia, deadzone)
if(v_desired - deadzone > v_actual)
    accel = torque / inertia;
elseif(v_desired + deadzone < v_actual)
    accel = -torque / inertia;
else
    accel = 0;
end

== matlab function OrientationAnimationModel/Orientation/Motor Output/MATLAB Function2 ==
  data: v_desired input; accel output; v_actual input; torque input; inertia input; deadzone input
function accel  = fcn(v_desired, v_actual, torque, inertia, deadzone)
if(v_desired - deadzone > v_actual)
    accel = torque / inertia;
elseif(v_desired + deadzone < v_actual)
    accel = -torque / inertia;
else
    accel = 0;
end

== matlab function OrientationAnimationModel/Orientation/RH Tait-Bryan ZY'X'' Inverse ==
  data: X input; psi output; Y input; theta output; phi output
function [psi, theta, phi] = fcn(X,Y)

% psi = heading
% theta = pitch
% phi = bank

psi = atan2(X(2),X(1));
theta = atan2(X(3),sqrt(X(2)^2 + X(1)^2));
if(-Y(1) * sin(psi) + Y(2) * cos(psi) > 1)
    n = 1;
elseif(-Y(1) * sin(psi) + Y(2) * cos(psi) < -1)
    n = -1;
else
    n = -Y(1) * sin(psi) + Y(2) * cos(psi);
end
if(Y(3) > 0)
    phi = acos(n);
else
    phi = -acos(n);
end

== matlab function OrientationAnimationModel/Gravity Model/Altitude ==
  data: x input; alt output; y input; z input
function alt = fcn(x, y, z)

alt = sqrt(x^2 + y^2 + z^2) - (6.3781*10^6);

== matlab function OrientationAnimationModel/Orientation/Magnetorquer Model/Dipole Vector ==
  data: x input; m_result output; m_dipole input
function m_result  = fcn(x,m_dipole)

m_result = [0;0;0];
mag = sqrt(x(1)^2 + x(2)^2 + x(3)^2);
m_result(1) = m_dipole * (x(1) / mag);
m_result(2) = m_dipole * (x(2) / mag);
m_result(3) = m_dipole * (x(3) / mag);

== matlab function OrientationAnimationModel/Orientation/Magnetorquer Model/Dipole Vector2 ==
  data: x input; m_result output; m_dipole input
function m_result  = fcn(x,m_dipole)

m_result = [0;0;0];
mag = sqrt(x(1)^2 + x(2)^2 + x(3)^2);
m_result(1) = m_dipole * (x(1) / mag);
m_result(2) = m_dipole * (x(2) / mag);
m_result(3) = m_dipole * (x(3) / mag);

== matlab function OrientationAnimationModel/Orientation/Animation Output/e2axis ==
  data: heading input; pitch input; roll input; vector output

function vector = e2axis(heading, pitch, roll)

eul = [heading -pitch roll];
coder.extrinsic('eul2rotm');
coder.extrinsic('rotm2axang');
rotm = eul2rotm(eul,'ZYX');
v = rotm2axang(rotm);
vector = [0;0;0;0];
vector(1) = v(1);
vector(2) = v(2);
vector(3) = v(3);
vector(4) = v(4);

end

== matlab function OrientationAnimationModel/Orientation/Magnetorquer Model/Magnetic Field Vector ==
  data: x input; B output; y input; z input
function B  = fcn(x,y,z)

B = [0;0;0];
q1 = 150; % bottom charge
q2 = 180; % top charge
r_earth = 6.3781e6;
inset = 2/3;
d_t = x^2 + y^2 + (z - r_earth * inset)^2; % distance squared from top charge to point
d_b = x^2 + y^2 + (z + r_earth * inset)^2; % distance squared from bottom charge to point

B(1) = (x) * (q1 / d_b - q2 / d_t);
B(2) = (y) * (q1 / d_b - q2 / d_t);
B(3) = (q1 / d_b) * (z + r_earth * inset) - (q1 / d_t) * (z - r_earth * inset);

== matlab function OrientationAnimationModel/Orientation/Animation Output/Anim Vector Creator ==
  data: mag_vec input; vec output
function vec = fcn(mag_vec)

cos_theta = mag_vec(3) / sqrt(mag_vec(1)^2+mag_vec(2)^2+mag_vec(3)^2);
theta = acos(cos_theta);
vec = [-mag_vec(2); mag_vec(1); 0; theta];
